simulink model "powersimACMC"  (Simulink 7.9)
settings: Solver=ode45  StartTime=0.0  StopTime=0.02  RelTol=1e-3
libraries: powerlib x11, simulink x1
settings Model: Creator=kidd  LastModifiedBy=jasonkidd
settings DebuggingCC: FcnCallInpInsideContextMsg=Use local settings
settings GRTTargetCC: CombineOutputUpdateFcns=off  GRTInterface=on

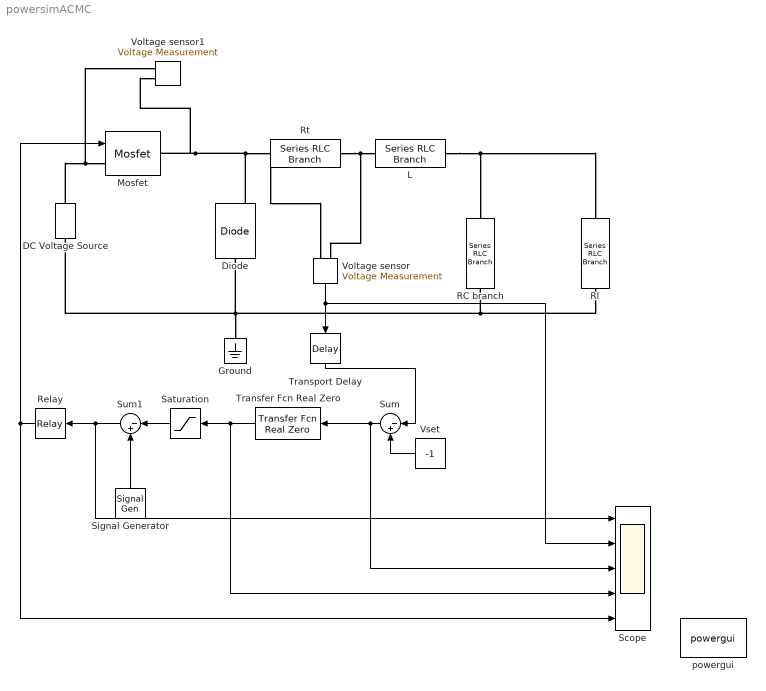
== system powersimACMC ==
  DC Voltage Source : powerlib/Electrical Sources/DC Voltage Source  Amplitude=30  Measurements=None
  Diode : powerlib/Power Electronics/Diode  Ron=0.001  Lon=0  Vf=0.8  IC=0  UseSnubber=off  Rs=500000  Cs=250e-9  Measurements=on
  Ground : powerlib/Elements/Ground  LConnTagsString=a
  L : powerlib/Elements/Series RLC Branch  LConnTagsString=__new0  RConnTagsString=__new0  BranchType=L  Resistance=1  Inductance=100e-6  SetiL0=off  InitialCurrent=0  Capacitance=1e-6  Setx0=off  InitialVoltage=0  Measurements=None
  Mosfet : powerlib/Power Electronics/Mosfet  Ron=0.1  Lon=0  Rd=0.01  Vfd=0  IC=0  Rs=1e8  Cs=inf  Measurements=off
  RC branch : powerlib/Elements/Series RLC Branch  LConnTagsString=__new0  RConnTagsString=__new0  BranchType=RC  Resistance=5e-3  Inductance=1e-3  SetiL0=off  InitialCurrent=0  Capacitance=1e-2  Setx0=off  InitialVoltage=0  Measurements=None
  Relay : Relay  OnOutputValue=5
  Rl : powerlib/Elements/Series RLC Branch  LConnTagsString=__new0  RConnTagsString=__new0  BranchType=R  Resistance=2  Inductance=1e-3  SetiL0=off  InitialCurrent=0  Capacitance=1e-6  Setx0=off  InitialVoltage=0  Measurements=None
  Rt : powerlib/Elements/Series RLC Branch  LConnTagsString=__new0  RConnTagsString=__new0  BranchType=R  Resistance=0.2  Inductance=1e-3  SetiL0=off  InitialCurrent=0  Capacitance=1e-6  Setx0=off  InitialVoltage=0  Measurements=None
  Saturation : Saturate  UpperLimit=1  ZeroCross=off
  Scope : Scope  NumInputPorts=5
      settings: TimeRange=0.004  YMin=-5~-0.01~-5~-5~-5  YMax=5~0.1~5~5~5
  Signal Generator : SignalGenerator  WaveForm=sawtooth  Amplitude=5  Frequency=100000
  Sum : Sum  Inputs=|-+
  Sum1 : Sum  Inputs=|-+
  Transfer Fcn Real Zero : simulink/Discrete/Transfer Fcn Real Zero  ZeroZ=0.5  ICPrevInput=0  InputProcessing=Inherited  DoSatur=off
  Transport Delay : TransportDelay  DelayTime=0.001
  Voltage sensor : powerlib/Measurements/Voltage Measurement  PhasorSimulation=off  OutputType=Complex  PSBequivalent=0
  Voltage sensor1 : powerlib/Measurements/Voltage Measurement  PhasorSimulation=off  OutputType=Complex  PSBequivalent=0
  Vset : Constant  Value=-1
  powergui : powerlib/powergui  Priority=1  SimulationMode=Continuous  SolverType=Tustin  SampleTime=50e-6  frequency=60  SPID=off  DisableSnubberDevices=off  DisableRonSwitches=off  DisableVfSwitches=off  SwTol=0  Interpol=off  DisplayEquations=off  FunctionMessages=off  frequencyindice=0  Pbase=100e6  ErrMax=1e-4  Iterations=50  UnitsV=kV  UnitsW=MW  echomessages=off  HookPort=off  EnableUseOfTLC=off  x0status=blocks  RestoreLinks=warning  ResistiveCurrentMeasurement=off  Ylog=off  Xlog=on  ShowGrid=off  save=off  variable=ZData  ZoomFFT=off  StartTime=0.0  cycles=1  DisplayStyle=1  FreqAxis=off  MaxFrequency=1000  frequencyindicesteady=1  display=off  methode=off
  wires:
  Sum1/1 -> Relay/1, Scope/1
  Voltage sensor/1 -> Transport Delay/1, Scope/2
  Transport Delay/1 -> Sum/1
  Transfer Fcn Real Zero/1 -> Saturation/1, Scope/4
  Relay/1 -> Mosfet/1, Scope/5
  Vset/1 -> Sum/2
  Sum/1 -> Transfer Fcn Real Zero/1, Scope/3
  Signal Generator/1 -> Sum1/2
  Saturation/1 -> Sum1/1
  connections:
  DC Voltage Source/RConn1 -- Mosfet/LConn1 -- Voltage sensor1/LConn1
  Diode/RConn1 -- Rt/RConn1 -- Voltage sensor/LConn1 -- Mosfet/RConn1 -- Voltage sensor1/LConn2
  L/RConn1 -- RC branch/RConn1 -- Rl/LConn1
  Rl/RConn1 -- RC branch/LConn1 -- Ground/LConn1 -- DC Voltage Source/LConn1 -- Diode/LConn1
  Rt/LConn1 -- L/LConn1 -- Voltage sensor/LConn2
